simulink model "Planta2"  (R2020a)
settings: Solver=VariableStepAuto  StartTime=0.0  StopTime=100  RelTol=1e-3
settings Model: Creator=Sergio  LastModifiedBy=Sergio

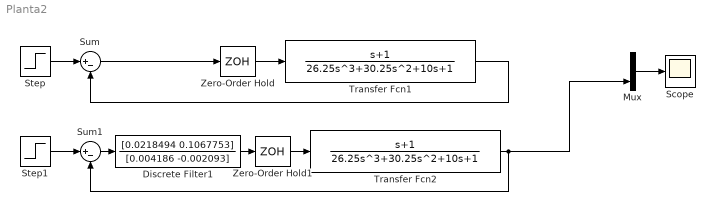
== system Planta2 ==
  Discrete Filter1 : DiscreteFilter  Numerator=[0.0218494 0.1067753]  Denominator=[0.004186 -0.002093]
  Mux : Mux  Inputs=2
  Scope : Scope
  Step : Step  Time=0  SampleTime=0
  Step1 : Step  Time=0  SampleTime=0
  Sum : Sum  Inputs=|+-
  Sum1 : Sum  Inputs=|+-
  Transfer Fcn1 : TransferFcn  Numerator=[1 1]  Denominator=[26.25 30.25 10 1]
  Transfer Fcn2 : TransferFcn  Numerator=[1 1]  Denominator=[26.25 30.25 10 1]
  Zero-Order Hold : ZeroOrderHold  SampleTime=0.2
  Zero-Order Hold1 : ZeroOrderHold  SampleTime=0.2
  wires:
  Transfer Fcn1/1 -> Sum/2
  Mux/1 -> Scope/1
  Step/1 -> Sum/1
  Zero-Order Hold/1 -> Transfer Fcn1/1
  Step1/1 -> Sum1/1
  Sum1/1 -> Discrete Filter1/1
  Zero-Order Hold1/1 -> Transfer Fcn2/1
  Transfer Fcn2/1 -> Mux/2, Sum1/2
  Discrete Filter1/1 -> Zero-Order Hold1/1
  Sum/1 -> Zero-Order Hold/1
